simulink subsystem "LeastCov_v2_adaptiveAlgorithm"  (R2022a)
settings: Solver=VariableStepAuto  StartTime=0.0  StopTime=10.0  RelTol=1e-3
libraries: simulink x2
settings Model: Creator=targi  LastModifiedBy=targi

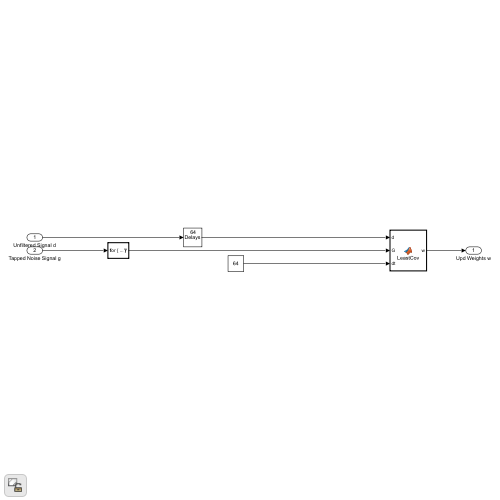
[thumbnail: Simulink's stored preview of the top-level diagram]
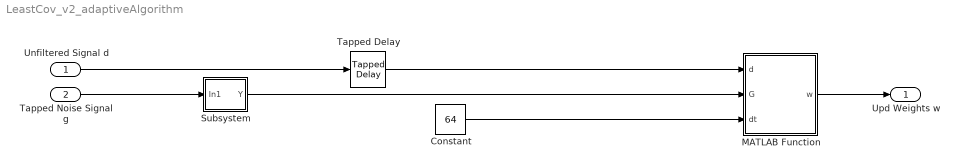
== system LeastCov_v2_adaptiveAlgorithm ==
  Unfiltered Signal d : Inport
  Tapped Noise Signal g : Inport  Port=2
  Constant : Constant  Value=64
  MATLAB Function : MATLAB Function  TreatAsAtomicUnit=on
  Subsystem : Subsystem
  Tapped Delay : simulink/Discrete/Tapped Delay  vinit=0.0  samptime=-1  NumDelays=64  DelayOrder=Oldest  includeCurrent=off
  Upd Weights w : Outport
  wires:
  Unfiltered Signal d/1 -> Tapped Delay/1
  MATLAB Function/1(w) -> Upd Weights w/1
  Tapped Delay/1 -> MATLAB Function/1(d)
  Constant/1 -> MATLAB Function/3(dt)
  Tapped Noise Signal g/1 -> Subsystem/1(In1)
  Subsystem/1(Y) -> MATLAB Function/2(G)

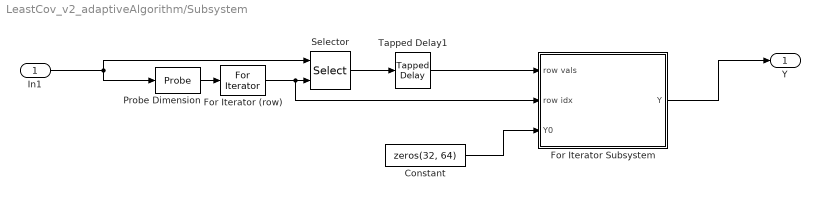
== system LeastCov_v2_adaptiveAlgorithm/Subsystem ==
  In1 : Inport
  Constant : Constant  Value=zeros(32, 64)
  For Iterator Subsystem : Subsystem  TreatAsAtomicUnit=on
  For Iterator (row) : ForIterator  IterationSource=external
  Probe Dimension : Probe  ProbeSampleTime=off  ProbeComplexSignal=off
  Selector : Selector  IndexOptions=Starting index (port)  Indices=[1 3]  OutputSizes=1
  Tapped Delay1 : simulink/Discrete/Tapped Delay  vinit=0.0  samptime=-1  NumDelays=64  DelayOrder=Oldest  includeCurrent=off
  Y : Outport
  wires:
  For Iterator Subsystem/1(Y) -> Y/1
  Constant/1 -> For Iterator Subsystem/3(Y0)
  Tapped Delay1/1 -> For Iterator Subsystem/1(row vals)
  For Iterator (row)/1 -> Selector/2, For Iterator Subsystem/2(row idx)
  Probe Dimension/1 -> For Iterator (row)/1
  In1/1 -> Selector/1, Probe Dimension/1
  Selector/1 -> Tapped Delay1/1

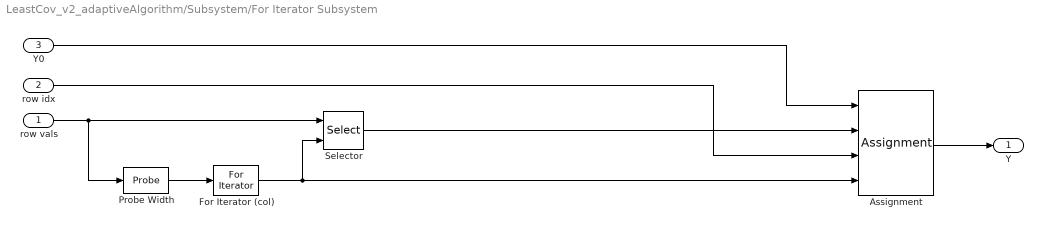
== system LeastCov_v2_adaptiveAlgorithm/Subsystem/For Iterator Subsystem ==
  row vals : Inport
  row idx : Inport  Port=2
  Y0 : Inport  Port=3
  Assignment : Assignment  NumberOfDimensions=2  DiagnosticForDimensions=Warning  IndexOptions=Index vector (port),Index vector (port)  Indices=1,1  OutputSizes=1,1
  For Iterator (col) : ForIterator  IterationSource=external
  Probe Width : Probe  ProbeSampleTime=off  ProbeComplexSignal=off
  Selector : Selector  IndexOptions=Index vector (port)  Indices=[1 3]  OutputSizes=1
  Y : Outport
  wires:
  Selector/1 -> Assignment/2
  Y0/1 -> Assignment/1
  row idx/1 -> Assignment/3
  For Iterator (col)/1 -> Assignment/4, Selector/2
  Probe Width/1 -> For Iterator (col)/1
  row vals/1 -> Selector/1, Probe Width/1
  Assignment/1 -> Y/1

== matlab function LeastCov_v2_adaptiveAlgorithm/MATLAB Function ==
  data: d input; w output; G input; dt input
function w = LeastCov(d, G, dt)

% time across the horizontal, weights down the vertical 

A = dt*G*d;
C = sum(G,2);
B = sum(d).*C;
D = dt*(sum(G.^2,2));

w = (A-B)./(2*(C-D));
